simulink model "series_hybrid_powertrain"  (R2022a)
settings: Solver=ode23tb  StartTime=0.0  StopTime=100  RelTol=1e-3
InitFcn:
  | m=1200;
  | c=.3;
  | frr=0.02;
  | g=9.81;
  | Cmax=24;
  | et=0.9;
  | i_f=3;
  | i1=3;
  | rw=.3;
undefined symbols (not defined in the file): C, J
libraries: autolibshared x1, slpidlib x1
settings Model: Creator=Kamyar  LastModifiedBy=harshkum5
settings SolverCC: AlgebraicLoopSolver=TrustRegion
settings DebuggingCC: UnconnectedInputMsg=warning  UnconnectedOutputMsg=warning  UnconnectedLineMsg=warning
settings RTWCC: DLArmComputeVersion=19.05

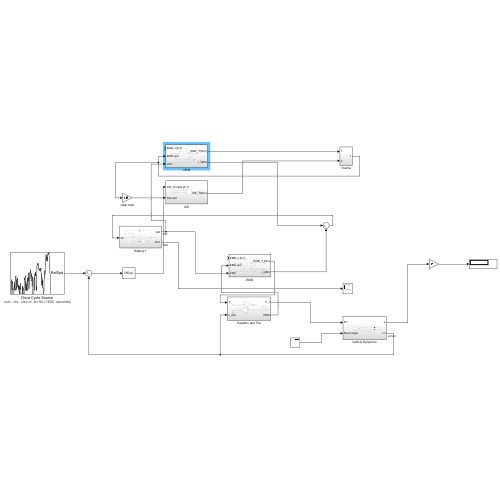
[thumbnail: Simulink's stored preview of the top-level diagram]
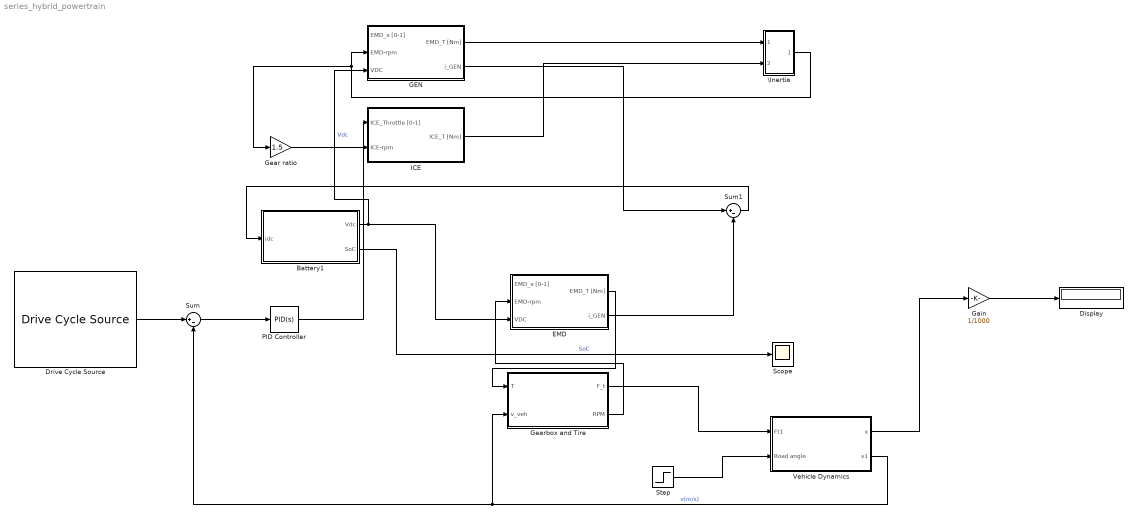
== system series_hybrid_powertrain ==
  Battery1 : Subsystem
  Display : Display
  Drive Cycle Source : autolibshared/Drive Cycle Source  cycleVar=.mat, .xls, .xlsx or .txt file  fileVar=C:\Users\harshkum5\Desktop\AVS\7. WLTP Class 3_Driving Cycle_v.xlsx  tfinal="1800  seconds"  cycleRepeat=off  outAccPort=off  outGearPort=off  gearList=No gear data  t_wot1=5  xdot_woto=0  xdot_wot1=30  t_wot2=20  xdot_wot2=0  t_wotend=30  srcUnit=m/s  outUnit=m/s  srcAccUnit=m/s/s  outAccUnit=m/s^2  dt=0  aMode=1  faultOption=off  velBnd=2  velBndUnit=mph  inUnit=m/s  timeBnd=1  failOption=off  stopSim=off  maxFaultCnt=10  maxFaultTime=2  maxTotFaultTime=15  traceOption=off  dtTrace=1  traceWindow=10  lastDCname=FTP75  lastOutUnit=mph  lastDT=0  lastTB=1  lastSB=2  forceCalcBound=off
      settings: SourceProductBaseCode=PW,DR,MT,VE
  EMD : Subsystem
  GEN : Subsystem
  Gain : Gain  Gain=1/1000
  Gear ratio : Gain  Gain=1.5
  Gearbox and Tire : Subsystem
  ICE : Subsystem
  PID Controller : slpidlib/PID Controller  Controller=PID  Form=Parallel  TimeDomain=Continuous-time  UseExternalTs=off  SampleTime=-1  IntegratorMethod=Forward Euler  FilterMethod=Forward Euler  ControllerParametersSource=internal  P=1  I=1  UseKiTs=off  D=0  N=100  UseFilter=on  TunerSelectOption=Transfer Function Based (PID Tuner App)  InitialConditionSource=internal  InitialConditionForIntegrator=0  InitialConditionForFilter=0  DifferentiatorICPrevScaledInput=0  ExternalReset=none  TrackingMode=off  Kt=1  LimitOutput=off  SatLimitsSource=internal  UpperSaturationLimit=inf  LowerSaturationLimit=-inf  LinearizeAsGain=on  AntiWindupMode=none  Kb=1  POutMin=[]  POutMax=[]  IOutMin=[]  IOutMax=[]  DOutMin=[]  DOutMax=[]  NOutMin=[]  NOutMax=[]  SumOutMin=[]  SumOutMax=[]  SaturationOutMin=[]  SaturationOutMax=[]  PParamMin=[]  PParamMax=[]  IParamMin=[]  IParamMax=[]  DParamMin=[]  DParamMax=[]  NParamMin=[]  NParamMax=[]  KbParamMin=[]  KbParamMax=[]  KtParamMin=[]  KtParamMax=[]  KbOutMin=[]  KbOutMax=[]  KtOutMin=[]  KtOutMax=[]  IntegratorOutMin=[]  IntegratorOutMax=[]  FilterOutMin=[]  FilterOutMax=[]  SumI1OutMin=[]  SumI1OutMax=[]  SumI2OutMin=[]  SumI2OutMax=[]  SumI3OutMin=[]  SumI3OutMax=[]  SumI4OutMin=[]  SumI4OutMax=[]  SumDOutMin=[]  SumDOutMax=[]  DifferentiatorOutMin=[]  DifferentiatorOutMax=[]  FilterDiffOutCoefMin=[]  FilterDiffOutCoefMax=[]  ReciprocalOutMin=[]  ReciprocalOutMax=[]  SumDenOutMin=[]  SumDenOutMax=[]  SumNumOutMin=[]  SumNumOutMax=[]  DivideOutMin=[]  DivideOutMax=[]  UdiffTsProdOutMin=[]  UdiffTsProdOutMax=[]  NTsProdOutMin=[]  NTsProdOutMax=[]  UintegralTsProdOutMin=[]  UintegralTsProdOutMax=[]  UngainTsProdOutMin=[]  UngainTsProdOutMax=[]  IntegratorContinuousStateAttributes=''  IntegratorStateMustResolveToSignalObject=off  IntegratorRTWStateStorageClass=Auto  FilterContinuousStateAttributes=''  FilterStateMustResolveToSignalObject=off  FilterRTWStateStorageClass=Auto  ParallelPVariant=InternalParameters  IdealPVariant=Disabled  IVariant=InternalParameters  DVariant=InternalParameters  IntegratorVariant=Continuous  SatVariant=Disabled  AWVariant=Passthrough  PCopyVariant=Disabled  TRVariant=Disabled  FdbkBlocksVariant=Forward  IdealPFdbkVariant=Disabled  SatFdbkVariant=Disabled  DerivativeFilterVariant=ContFilter  NVariant=InternalParameters  NCopyVariant=Disabled  FilterICVariant=InternalICsFilter  IntegratorICVariant=InternalICs  ExternalResetVariant=Disabled  TRSumVariant=Passthrough  SumFdbkVariant=Disabled  SumVariant=Sum_PID  TsampFilterVariant=InternalTs  TsampNgainVariant=Passthrough  TsampIntegralVariant=Passthrough  ExternalSaturationOutDataTypeStr=Inherit: Same as second input  aMode=0
  Scope : Scope
  Step : Step  SampleTime=0
  Sum : Sum  Inputs=|+-
  Sum1 : Sum  Inputs=|+-
  Vehicle Dynamics : Subsystem
  \Inertia : Subsystem
  wires:
  Gear ratio/1 -> ICE/2(ICE-rpm)
  EMD/2(i_GEN) -> Sum1/2
  GEN/2(i_GEN) -> Sum1/1
  Battery1/1(Vdc) -> GEN/3(VDC), EMD/3(VDC)  "Vdc"
  Sum1/1 -> Battery1/1(idc)
  Battery1/2(SoC) -> Scope/1  "SoC"
  \Inertia/1(Out1) -> Gear ratio/1, GEN/2(EMD-rpm)
  GEN/1(EMD_T [Nm]) -> \Inertia/1(In1)
  ICE/1(ICE_T [Nm]) -> \Inertia/2(In2)
  Gearbox and Tire/2(RPM) -> EMD/2(EMD-rpm)
  Gearbox and Tire/1(F_t) -> Vehicle Dynamics/1(Ft1)
  Step/1 -> Vehicle Dynamics/2(Road angle)
  Vehicle Dynamics/1(x) -> Gain/1
  Gain/1 -> Display/1
  Vehicle Dynamics/2(v1) -> Sum/2, Gearbox and Tire/2(v_veh)  "v(m/s)"
  EMD/1(EMD_T [Nm]) -> Gearbox and Tire/1(T)
  Drive Cycle Source/1 -> Sum/1
  Sum/1 -> PID Controller/1
  PID Controller/1 -> ICE/1(ICE_Throttle [0-1])

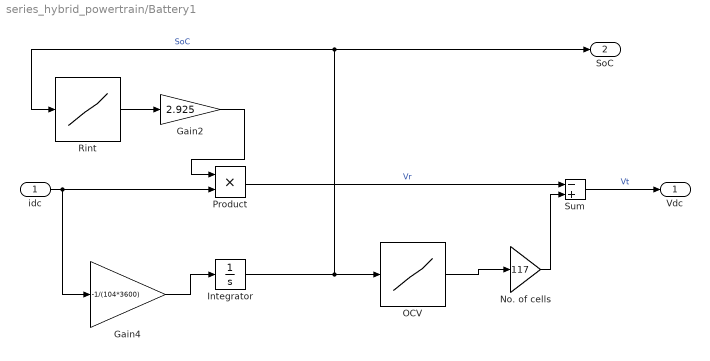
== system series_hybrid_powertrain/Battery1 ==
  idc : Inport
  Gain2 : Gain  Gain=2.925
  Gain4 : Gain  Gain=-1/(104*3600)
  Integrator : Integrator  InitialCondition=1
  No. of cells : Gain  Gain=117
  OCV : Lookup_n-D  NumberOfTableDimensions=1  BreakpointsForDimension1=[0;0.020877;0.038336;0.063;0.088708;0.117522;0.153557;0.191659;0.253454;0.40178;0.551119;0.700468;0.819937;0.906457;0.960023;0.980623;0.994005;0.998104;1]  Table=[2.5;2.701493;2.840939;2.997836;3.119894;3.207123;3.272604;3.325027;3.386261;3.495764;3.64447;3.771399;3.898204;3.968251;3.998962;4.01647;4.047013;4.099295;4.2]  InternalRulePriority=Speed  RndMeth=Simplest
  Product : Product
  Rint : Lookup_n-D  NumberOfTableDimensions=1  BreakpointsForDimension1=|  Table=|  InternalRulePriority=Speed  RndMeth=Simplest
      BreakpointsForDimension1=|
      | [0
      | 0.041223404
      | 0.099734043
      | 0.200797872
      | 0.39893617
      | 0.599734043
      | 0.800531915
      | 1
      | ]
      Table=|
      | [0.135819057
      | 0.128988915
      | 0.091367148
      | 0.079722316
      | 0.069868996
      | 0.070764752
      | 0.074347777
      | 0.057328407
      | ]
  Sum : Sum  Inputs=-+
  Vdc : Outport
  SoC : Outport  Port=2
  wires:
  Sum/1 -> Vdc/1  "Vt"
  No. of cells/1 -> Sum/2
  Product/1 -> Sum/1  "Vr"
  OCV/1 -> No. of cells/1
  Rint/1 -> Gain2/1
  Gain2/1 -> Product/1
  idc/1 -> Gain4/1, Product/2
  Integrator/1 -> SoC/1, Rint/1, OCV/1  "SoC"
  Gain4/1 -> Integrator/1

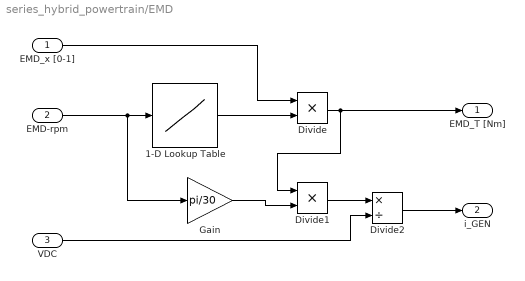
== system series_hybrid_powertrain/EMD ==
  EMD_x [0-1] : Inport
  EMD-rpm : Inport  Port=2
  VDC : Inport  Port=3
  1-D Lookup Table : Lookup_n-D  NumberOfTableDimensions=1  BreakpointsForDimension1=[0;962.0253;2126.582;3341.772;4607.595;5240.506;5822.785;6607.595;7594.937;8329.114;9316.456;10582.28;11949.37;13240.51;14000]  Table=[340.1599;339.6231;339.6712;339.1428;327.0423;302.7629;280.7962;250.7361;221.8417;202.1961;180.8249;153.0995;130.5865;112.1214;102.3148]  InternalRulePriority=Speed  RndMeth=Simplest
  Divide : Product
  Divide1 : Product
  Divide2 : Product  Inputs=*/
  Gain : Gain  Gain=pi/30
  EMD_T [Nm] : Outport
  i_GEN : Outport  Port=2
  wires:
  EMD-rpm/1 -> Gain/1, 1-D Lookup Table/1
  1-D Lookup Table/1 -> Divide/2
  EMD_x [0-1]/1 -> Divide/1
  Divide/1 -> Divide1/1, EMD_T [Nm]/1
  Divide1/1 -> Divide2/1
  Divide2/1 -> i_GEN/1
  VDC/1 -> Divide2/2
  Gain/1 -> Divide1/2

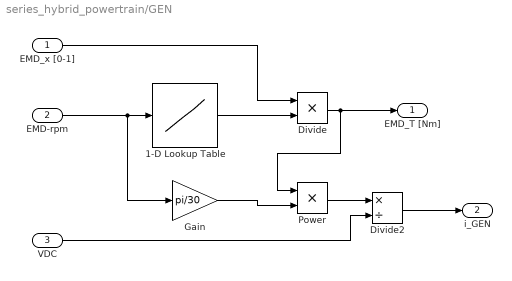
== system series_hybrid_powertrain/GEN ==
  EMD_x [0-1] : Inport
  EMD-rpm : Inport  Port=2
  VDC : Inport  Port=3
  1-D Lookup Table : Lookup_n-D  NumberOfTableDimensions=1  BreakpointsForDimension1=[0;962.0253;2126.582;3341.772;4607.595;5240.506;5822.785;6607.595;7594.937;8329.114;9316.456;10582.28;11949.37;13240.51;14000]  Table=[340.1599;339.6231;339.6712;339.1428;327.0423;302.7629;280.7962;250.7361;221.8417;202.1961;180.8249;153.0995;130.5865;112.1214;102.3148]  InternalRulePriority=Speed  RndMeth=Simplest
  Divide : Product
  Divide2 : Product  Inputs=*/
  Gain : Gain  Gain=pi/30
  Power : Product
  EMD_T [Nm] : Outport
  i_GEN : Outport  Port=2
  wires:
  EMD-rpm/1 -> Gain/1, 1-D Lookup Table/1
  1-D Lookup Table/1 -> Divide/2
  EMD_x [0-1]/1 -> Divide/1
  Divide/1 -> Power/1, EMD_T [Nm]/1
  Power/1 -> Divide2/1
  VDC/1 -> Divide2/2
  Divide2/1 -> i_GEN/1
  Gain/1 -> Power/2

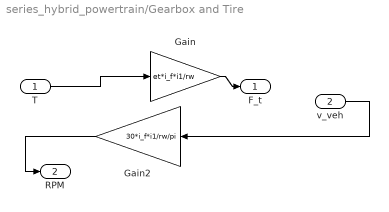
== system series_hybrid_powertrain/Gearbox and Tire ==
  T : Inport
  v_veh : Inport  Port=2
  Gain : Gain  Gain=et*i_f*i1/rw
  Gain2 : Gain  Gain=30*i_f*i1/rw/pi
  F_t : Outport
  RPM : Outport  Port=2
  wires:
  Gain2/1 -> RPM/1
  T/1 -> Gain/1
  v_veh/1 -> Gain2/1
  Gain/1 -> F_t/1

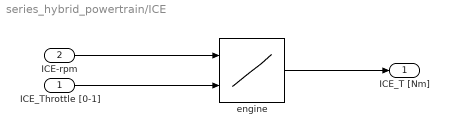
== system series_hybrid_powertrain/ICE ==
  ICE_Throttle [0-1] : Inport
  ICE-rpm : Inport  Port=2
  engine : Lookup_n-D  BreakpointsForDimension1=1000:1000:6000  BreakpointsForDimension2=0:.25:1  Table=|  InternalRulePriority=Speed  RndMeth=Simplest
      | [0.1	120	200	234	270
      | 0.1	129.2307692	215.3846154	252	300
      | 0.1	120	200	252	315
      | 0.1	50	160	243	310
      | 0.1	0	100	180	250
      | 0.1	0	0	90	180
      | ]
      settings: InputPortMap=u0,u1
  ICE_T [Nm] : Outport
  wires:
  engine/1 -> ICE_T [Nm]/1
  ICE-rpm/1 -> engine/1
  ICE_Throttle [0-1]/1 -> engine/2

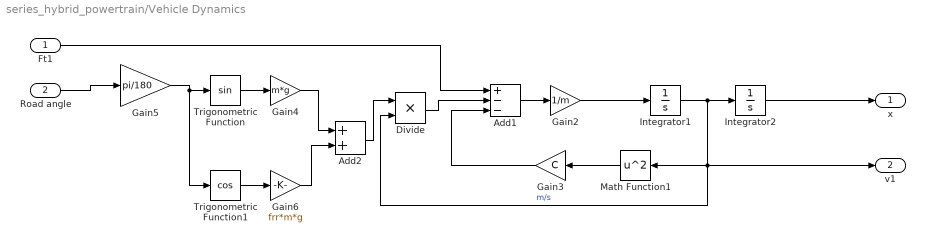
== system series_hybrid_powertrain/Vehicle Dynamics ==
  Ft1 : Inport
  Road angle : Inport  Port=2
  Add1 : Sum  Inputs=+--
  Add2 : Sum
  Divide : Product
  Gain2 : Gain  Gain=1/m
  Gain3 : Gain  Gain=C
  Gain4 : Gain  Gain=m*g
  Gain5 : Gain  Gain=pi/180
  Gain6 : Gain  Gain=frr*m*g
  Integrator1 : Integrator
  Integrator2 : Integrator
  Math Function1 : Math  Operator=square
  Trigonometric Function : Trigonometry
  Trigonometric Function1 : Trigonometry  Operator=cos
  x : Outport
  v1 : Outport  Port=2
  wires:
  Trigonometric Function/1 -> Gain4/1
  Integrator2/1 -> x/1
  Add2/1 -> Divide/1
  Add1/1 -> Gain2/1
  Gain5/1 -> Trigonometric Function1/1, Trigonometric Function/1
  Gain2/1 -> Integrator1/1
  Ft1/1 -> Add1/1
  Road angle/1 -> Gain5/1
  Integrator1/1 -> Divide/2, v1/1, Math Function1/1, Integrator2/1  "m/s"
  Gain6/1 -> Add2/2
  Gain4/1 -> Add2/1
  Math Function1/1 -> Gain3/1
  Gain3/1 -> Add1/3
  Trigonometric Function1/1 -> Gain6/1
  Divide/1 -> Add1/2

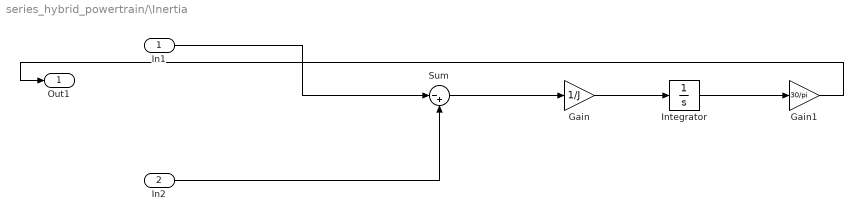
== system series_hybrid_powertrain/\Inertia ==
  In1 : Inport
  In2 : Inport  Port=2
  Gain : Gain  Gain=1/J
  Gain1 : Gain  Gain=30/pi
  Integrator : Integrator
  Sum : Sum  Inputs=|-+
  Out1 : Outport
  wires:
  Sum/1 -> Gain/1
  Gain/1 -> Integrator/1
  Integrator/1 -> Gain1/1
  In2/1 -> Sum/2
  In1/1 -> Sum/1
  Gain1/1 -> Out1/1
